simulink model "BPSK_Model"  (R2014a)
settings: Solver=ode45  StartTime=0.0  StopTime=50  RelTol=1e-3  AbsTol=1e-6
values from neighbouring files (symbols this model uses):
  G = Simulink.Parameter(5)    [BPSK.m]
  N_0 = Simulink.Parameter(N0_vals(i))    [BPSK.m]
libraries: commchan3 x1, commsink2 x1, commfilt2 x1, commanapbnd3 x1, commrandsrc2 x1, dspsrcs4 x1
settings Model: Creator=COOLSAM  LastModifiedBy=COOLSAM

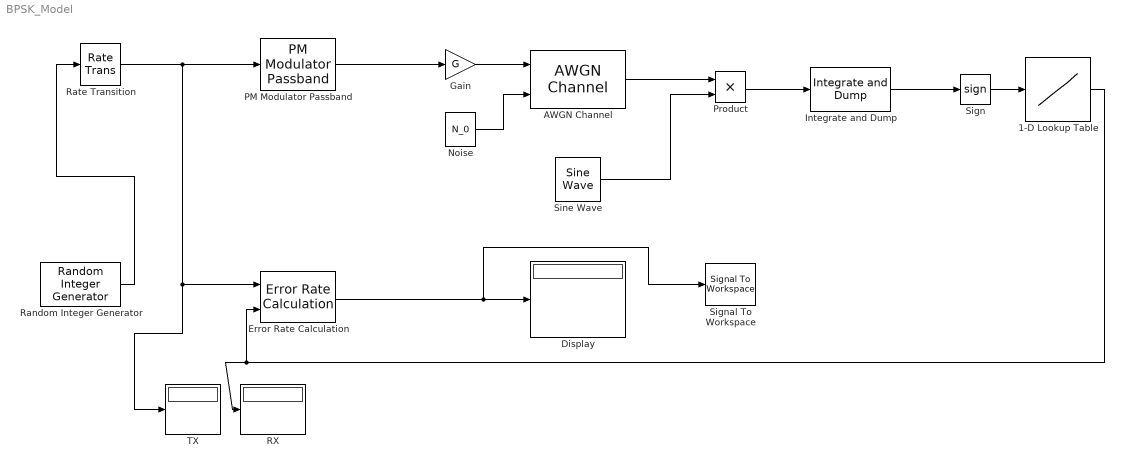
== system BPSK_Model ==
  1-D Lookup Table : Lookup_n-D  NumberOfTableDimensions=1  BreakpointsForDimension1=[-1 0 1]  Table=[-1 0 1]  InternalRulePriority=Speed  RndMeth=Simplest  InputSameDT=on
  AWGN Channel : commchan3/AWGN Channel  InputProcessing=Columns as channels (frame based)  seed=67  noiseMode=Variance from port  EbNodB=1  EsNodB=10  SNRdB=10  bitsPerSym=1  Ps=1  Tsym=1  variance=10
  Display : Display
  Error Rate Calculation : commsink2/Error Rate Calculation  N=0  st_delay=0  cp_mode=Entire frame  subframe=[]  PMode=Port  WsName=ErrorVec  RsMode2=off  stop=off  numErr=100  maxBits=1e6
  Gain : Gain  Gain=G  OutDataTypeStr=double  SampleTime=1e-3
  Integrate and Dump : commfilt2/Integrate and Dump  obssamples=4  offsetsamples=0  nodump=off  roundingMode=Floor  overflowMode=off
  Noise : Constant  Value=N_0  SampleTime=1e-3
  PM Modulator Passband : commanapbnd3/PM Modulator Passband  Fc=40e3  Ph=pi  Kc=pi
  Product : Product  OutDataTypeStr=double  RndMeth=Nearest
  RX : Display
  Random Integer Generator : commrandsrc2/Random Integer Generator  mul=2  seed=67  Ts=1e-3  frameBased=off  sampPerFrame=1  orient=on  outDataType=double
  Rate Transition : RateTransition  OutPortSampleTimeOpt=Multiple of input port sample time
  Sign : Signum  SampleTime=0.001
  Signal To Workspace : SignalToWorkspace  VariableName=Pb  SaveFormat=Structure With Time
      settings: CopyFcn=dspblkcopystw(gcbh);
  Sine Wave : dspsrcs4/Sine Wave  Amplitude=1  Frequency=100  Phase=pi  SampleMode=Discrete  OutComplex=Real  CompMethod=Trigonometric fcn  TableSize=Speed  SampleTime=1e-3  SamplesPerFrame=1  ResetState=Restart at time zero  dataType=double  wordLen=16  udDataType=sfix(16)  fracBitsMode=Best precision  numFracBits=15  OutDataTypeStr=double  LastOutDataTypeStr=double
  TX : Display
  wires:
  Error Rate Calculation/1 -> Signal To Workspace/1, Display/1
  Random Integer Generator/1 -> Rate Transition/1
  Rate Transition/1 -> TX/1, Error Rate Calculation/1, PM Modulator Passband/1
  PM Modulator Passband/1 -> Gain/1
  Gain/1 -> AWGN Channel/1
  AWGN Channel/1 -> Product/1
  Sine Wave/1 -> Product/2
  Product/1 -> Integrate and Dump/1
  1-D Lookup Table/1 -> RX/1, Error Rate Calculation/2
  Integrate and Dump/1 -> Sign/1
  Sign/1 -> 1-D Lookup Table/1
  Noise/1 -> AWGN Channel/2
